simulink model "posFuzzy"  (R2015a)
settings: Solver=ode45  SolverMode=SingleTasking  StartTime=0.0  StopTime=3  RelTol=1e-3
libraries: simulink x5, fuzblock x4, simulink_extras x3
settings Model: CovMetricSettings=dwe  CovHtmlReporting=off  covSaveCumulativeToWorkspaceVar=off  CovSaveSingleToWorkspaceVar=off  CovExternalEMLEnable=on  Creator=brand  LastModifiedBy=brand
settings DataIOCC: LimitDataPoints=off  SaveFormat=Dataset
settings DebuggingCC: SFUnexpectedBacktrackingDiag=error  SFNoUnconditionalDefaultTransitionDiag=error
settings HardwareCC: ProdBitPerPointer=64  ProdLargestAtomicFloat=Float  ProdIntDivRoundTo=Zero  ProdEndianess=LittleEndian  ProdHWDeviceType=Specified
settings ModelReferenceCC: PropagateSignalLabelsOutOfModel=on
settings GRTTargetCC: TargetLangStandard=C99 (ISO)  GeneratePreprocessorConditionals=Use local settings

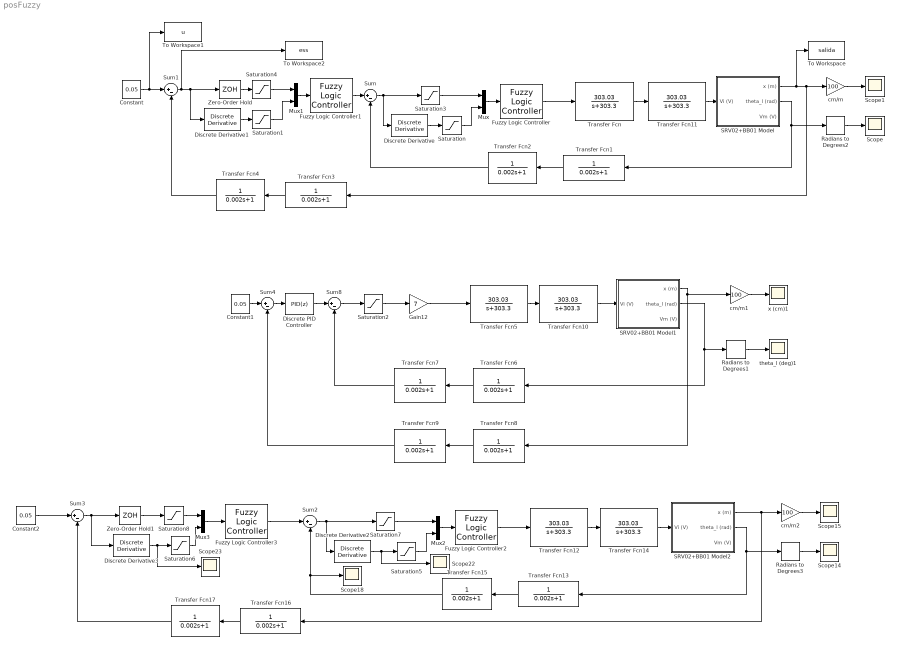
== system posFuzzy ==
  Constant : Constant  Value=0.05
  Constant1 : Constant  Value=0.05
  Constant2 : Constant  Value=0.05
  Discrete Derivative{,1..3} (4 alike) : simulink/Discrete/Discrete Derivative  gainval=1.0  ICPrevScaledInput=0.0  OutMin=[]  OutMax=[]  OutDataType=fixdt(1, 16)  OutScaling=2^-10  DoSatur=off
  Discrete PID Controller : simulink/Continuous/PID Controller  Controller=PID  TimeDomain=Discrete-time  SampleTime=12e-3  IntegratorMethod=Forward Euler  FilterMethod=Forward Euler  Form=Parallel  UseFilter=on  ControllerParametersSource=internal  P=12  I=0  D=6.5  N=100  InitialConditionSource=internal  InitialConditionForIntegrator=0  InitialConditionForFilter=0  ExternalReset=none  LimitOutput=off  UpperSaturationLimit=inf  LowerSaturationLimit=-inf  LinearizeAsGain=off  AntiWindupMode=none  Kb=1  TrackingMode=off  Kt=1  PParamMin=[]  PParamMax=[]  IParamMin=[]  IParamMax=[]  DParamMin=[]  DParamMax=[]  NParamMin=[]  NParamMax=[]  KbParamMin=[]  KbParamMax=[]  KtParamMin=[]  KtParamMax=[]  POutMin=[]  POutMax=[]  IOutMin=[]  IOutMax=[]  DOutMin=[]  DOutMax=[]  NOutMin=[]  NOutMax=[]  KbOutMin=[]  KbOutMax=[]  KtOutMin=[]  KtOutMax=[]  IntegratorOutMin=[]  IntegratorOutMax=[]  FilterOutMin=[]  FilterOutMax=[]  SumOutMin=[]  SumOutMax=[]  SumI1OutMin=[]  SumI1OutMax=[]  SumI2OutMin=[]  SumI2OutMax=[]  SumI3OutMin=[]  SumI3OutMax=[]  SumDOutMin=[]  SumDOutMax=[]  SaturationOutMin=[]  SaturationOutMax=[]  IntegratorContinuousStateAttributes=''  IntegratorStateMustResolveToSignalObject=off  IntegratorRTWStateStorageClass=Auto  FilterContinuousStateAttributes=''  FilterStateMustResolveToSignalObject=off  FilterRTWStateStorageClass=Auto  DifferentiatorICPrevScaledInput=0  DifferentiatorOutMin=[]  DifferentiatorOutMax=[]
  Fuzzy Logic Controller : fuzblock/Fuzzy Logic  Controller  FIS=angulov6unicamf
  Fuzzy Logic Controller1 : fuzblock/Fuzzy Logic  Controller  FIS=posicion8unicamf
  Fuzzy Logic Controller2 : fuzblock/Fuzzy Logic  Controller  FIS=angulov6unicamf
  Fuzzy Logic Controller3 : fuzblock/Fuzzy Logic  Controller  FIS=optipos3h
  Gain12 : Gain  Gain=7
  Mux{,1..3} (4 alike) : Mux  Inputs=2
  Radians to Degrees1 : simulink_extras/Transformations/Radians to Degrees
  Radians to Degrees2 : simulink_extras/Transformations/Radians to Degrees
  Radians to Degrees3 : simulink_extras/Transformations/Radians to Degrees
  SRV02+BB01 Model : Subsystem
  SRV02+BB01 Model1 : Subsystem
  SRV02+BB01 Model2 : Subsystem
  Saturation : Saturate  UpperLimit=5  LowerLimit=-5
  Saturation1 : Saturate  UpperLimit=20  LowerLimit=-20
  Saturation2 : Saturate  UpperLimit=0.76  LowerLimit=-0.76
  Saturation3 : Saturate  UpperLimit=0.785  LowerLimit=-0.785
  Saturation4 : Saturate  UpperLimit=0.2  LowerLimit=-0.2
  Saturation5 : Saturate  UpperLimit=5  LowerLimit=-5
  Saturation6 : Saturate  UpperLimit=20  LowerLimit=-20
  Saturation7 : Saturate  UpperLimit=0.785  LowerLimit=-0.785
  Saturation8 : Saturate  UpperLimit=0.2  LowerLimit=-0.2
  Scope{,1,14..15,18,22..23} (7 alike) : Scope
      Scope settings: TimeRange=auto  MaxDataPoints=5000  SaveToWorkspace=off  SaveName=ScopeData  YMin=-21.83998  YMax=37.02972  SampleTime=-1
      Scope1 settings: TimeRange=auto  MaxDataPoints=5000  SaveName=difuso  YMin=-0.64374  YMax=5.79369  SampleTime=-1  DataFormat=Array
      Scope14 settings: TimeRange=auto  MaxDataPoints=5000  SaveToWorkspace=off  SaveName=ScopeData6  YMin=-21.83998  YMax=37.02972  SampleTime=-1
      Scope15 settings: TimeRange=auto  MaxDataPoints=5000  SaveName=optifuzzy  YMin=-0.63086  YMax=5.67771  SampleTime=-1  DataFormat=Array
      Scope18 settings: TimeRange=auto  MaxDataPoints=5000  SaveToWorkspace=off  SaveName=ScopeData9  YMin=-0.41326  YMax=0.50458  SampleTime=-1
      Scope22 settings: TimeRange=auto  MaxDataPoints=5000  SaveToWorkspace=off  SaveName=ScopeData13  YMin=-11.56987  YMax=45.64384  SampleTime=-1
      Scope23 settings: TimeRange=auto  MaxDataPoints=5000  SaveToWorkspace=off  SaveName=ScopeData14  YMin=-0.00059  YMax=-0.00038  SampleTime=-1
  Sum{,1..4,8} (6 alike) : Sum  Inputs=|+-
  To Workspace : ToWorkspace  VariableName=salida  SaveFormat=Structure With Time  SampleTime=-1
  To Workspace1 : ToWorkspace  VariableName=u  SampleTime=-1
  To Workspace2 : ToWorkspace  VariableName=ess  SampleTime=-1
  Transfer Fcn{,5,10..12,14} (6 alike) : TransferFcn  Numerator=[303.03]  Denominator=[1 303.3]
  Transfer Fcn{1..4,6..9,13,15..17} (12 alike) : TransferFcn  Denominator=[0.002 1]
  Zero-Order Hold : ZeroOrderHold  SampleTime=12e-3
  Zero-Order Hold1 : ZeroOrderHold  SampleTime=12e-3
  cm/m : Gain  Gain=100
  cm/m1 : Gain  Gain=100
  cm/m2 : Gain  Gain=100
  theta_l (deg)1 : Scope
      settings: TimeRange=0.2  MaxDataPoints=5000  SaveName=ScopeData8  YMin=-25.81025  YMax=4.78166  SampleTime=-1  DataFormat=Array
  x (cm)1 : Scope
      settings: TimeRange=10  MaxDataPoints=5000  SaveName=convencional  YMin=-0.70041  YMax=6.30365  SampleTime=-1  DataFormat=Array
  wires:
  Mux/1 -> Fuzzy Logic Controller/1
  Sum/1 -> Saturation3/1, Discrete Derivative/1
  Fuzzy Logic Controller/1 -> Transfer Fcn/1
  Transfer Fcn1/1 -> Transfer Fcn2/1
  SRV02+BB01 Model/2(theta_l (rad)) -> Radians to Degrees2/1, Transfer Fcn1/1
  Radians to Degrees2/1 -> Scope/1
  Fuzzy Logic Controller1/1 -> Sum/1
  Transfer Fcn3/1 -> Transfer Fcn4/1
  Transfer Fcn4/1 -> Sum1/2
  Zero-Order Hold/1 -> Saturation4/1
  Mux1/1 -> Fuzzy Logic Controller1/1
  Constant/1 -> To Workspace1/1, Sum1/1
  Discrete Derivative/1 -> Saturation/1
  Saturation/1 -> Mux/2
  Discrete Derivative1/1 -> Saturation1/1
  Saturation1/1 -> Mux1/2
  Saturation4/1 -> Mux1/1
  Transfer Fcn8/1 -> Transfer Fcn9/1
  SRV02+BB01 Model1/2(theta_l (rad)) -> Radians to Degrees1/1, Transfer Fcn6/1
  Sum8/1 -> Saturation2/1
  Saturation2/1 -> Gain12/1
  Sum4/1 -> Discrete PID Controller/1
  Constant1/1 -> Sum4/1
  Discrete PID Controller/1 -> Sum8/1
  Radians to Degrees1/1 -> theta_l (deg)1/1
  Gain12/1 -> Transfer Fcn5/1
  Transfer Fcn7/1 -> Sum8/2
  Transfer Fcn9/1 -> Sum4/2
  Transfer Fcn6/1 -> Transfer Fcn7/1
  SRV02+BB01 Model1/1(x (m)) -> cm/m1/1, Transfer Fcn8/1
  cm/m1/1 -> x (cm)1/1
  Transfer Fcn5/1 -> Transfer Fcn10/1
  Transfer Fcn10/1 -> SRV02+BB01 Model1/1(Vi (V))
  Transfer Fcn/1 -> Transfer Fcn11/1
  Saturation3/1 -> Mux/1
  Transfer Fcn11/1 -> SRV02+BB01 Model/1(Vi (V))
  Transfer Fcn2/1 -> Sum/2
  Transfer Fcn15/1 -> Sum2/2, Scope18/1
  Transfer Fcn14/1 -> SRV02+BB01 Model2/1(Vi (V))
  Saturation7/1 -> Mux2/1
  Transfer Fcn12/1 -> Transfer Fcn14/1
  Saturation8/1 -> Mux3/1
  cm/m2/1 -> Scope15/1
  Saturation6/1 -> Mux3/2
  Discrete Derivative3/1 -> Saturation6/1, Scope23/1
  Saturation5/1 -> Mux2/2
  Discrete Derivative2/1 -> Saturation5/1, Scope22/1
  Constant2/1 -> Sum3/1
  Mux3/1 -> Fuzzy Logic Controller3/1
  Zero-Order Hold1/1 -> Saturation8/1
  Transfer Fcn17/1 -> Sum3/2
  Sum3/1 -> Zero-Order Hold1/1, Discrete Derivative3/1
  SRV02+BB01 Model2/1(x (m)) -> Transfer Fcn16/1, cm/m2/1
  Fuzzy Logic Controller3/1 -> Sum2/1
  Radians to Degrees3/1 -> Scope14/1
  SRV02+BB01 Model2/2(theta_l (rad)) -> Transfer Fcn13/1, Radians to Degrees3/1
  Transfer Fcn13/1 -> Transfer Fcn15/1
  Fuzzy Logic Controller2/1 -> Transfer Fcn12/1
  Sum2/1 -> Discrete Derivative2/1, Saturation7/1
  Mux2/1 -> Fuzzy Logic Controller2/1
  Transfer Fcn16/1 -> Transfer Fcn17/1
  cm/m/1 -> Scope1/1
  Sum1/1 -> To Workspace2/1, Discrete Derivative1/1, Zero-Order Hold/1
  SRV02+BB01 Model/1(x (m)) -> To Workspace/1, cm/m/1, Transfer Fcn3/1

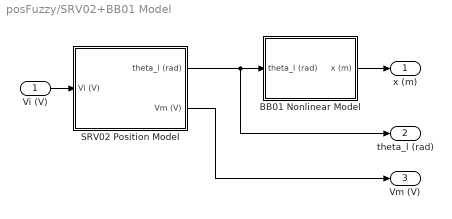
== system posFuzzy/SRV02+BB01 Model ==
  Vi (V) : Inport
  BB01 Nonlinear Model : Subsystem
  SRV02 Position Model : Subsystem
  x (m) : Outport
  theta_l (rad) : Outport  Port=2
  Vm (V) : Outport  Port=3
  wires:
  SRV02 Position Model/1(theta_l (rad)) -> BB01 Nonlinear Model/1(theta_l (rad)), theta_l (rad)/1
  BB01 Nonlinear Model/1(x (m)) -> x (m)/1
  Vi (V)/1 -> SRV02 Position Model/1(Vi (V))
  SRV02 Position Model/2(Vm (V)) -> Vm (V)/1

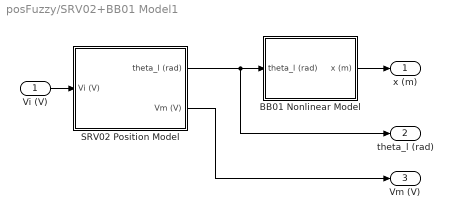
== system posFuzzy/SRV02+BB01 Model1 ==
  Vi (V) : Inport
  BB01 Nonlinear Model : Subsystem
  SRV02 Position Model : Subsystem
  x (m) : Outport
  theta_l (rad) : Outport  Port=2
  Vm (V) : Outport  Port=3
  wires:
  SRV02 Position Model/1(theta_l (rad)) -> BB01 Nonlinear Model/1(theta_l (rad)), theta_l (rad)/1
  BB01 Nonlinear Model/1(x (m)) -> x (m)/1
  Vi (V)/1 -> SRV02 Position Model/1(Vi (V))
  SRV02 Position Model/2(Vm (V)) -> Vm (V)/1

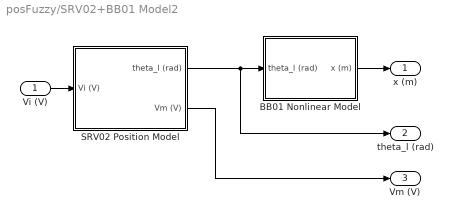
== system posFuzzy/SRV02+BB01 Model2 ==
  Vi (V) : Inport
  BB01 Nonlinear Model : Subsystem
  SRV02 Position Model : Subsystem
  x (m) : Outport
  theta_l (rad) : Outport  Port=2
  Vm (V) : Outport  Port=3
  wires:
  SRV02 Position Model/2(Vm (V)) -> Vm (V)/1
  Vi (V)/1 -> SRV02 Position Model/1(Vi (V))
  BB01 Nonlinear Model/1(x (m)) -> x (m)/1
  SRV02 Position Model/1(theta_l (rad)) -> theta_l (rad)/1, BB01 Nonlinear Model/1(theta_l (rad))

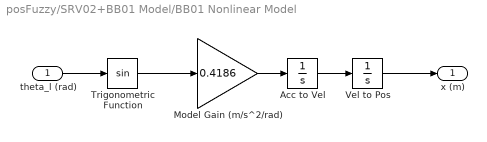
== system posFuzzy/SRV02+BB01 Model/BB01 Nonlinear Model ==
  theta_l (rad) : Inport
  Acc to Vel : Integrator
  Model Gain (m/s^2/rad) : Gain  Gain=0.4186
  Trigonometric Function : Trigonometry
  Vel to Pos : Integrator
  x (m) : Outport
  wires:
  theta_l (rad)/1 -> Trigonometric Function/1
  Vel to Pos/1 -> x (m)/1
  Model Gain (m/s^2/rad)/1 -> Acc to Vel/1
  Acc to Vel/1 -> Vel to Pos/1
  Trigonometric Function/1 -> Model Gain (m/s^2/rad)/1

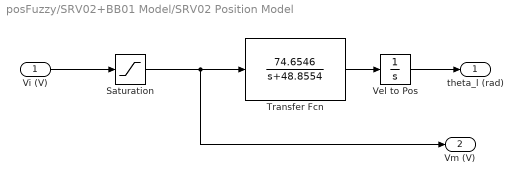
== system posFuzzy/SRV02+BB01 Model/SRV02 Position Model ==
  Vi (V) : Inport
  Saturation : Saturate  UpperLimit=5  LowerLimit=-5
  Transfer Fcn : TransferFcn  Numerator=[74.6546]  Denominator=[1 48.8554]
  Vel to Pos : Integrator
  theta_l (rad) : Outport
  Vm (V) : Outport  Port=2
  wires:
  Transfer Fcn/1 -> Vel to Pos/1
  Vel to Pos/1 -> theta_l (rad)/1
  Saturation/1 -> Vm (V)/1, Transfer Fcn/1
  Vi (V)/1 -> Saturation/1

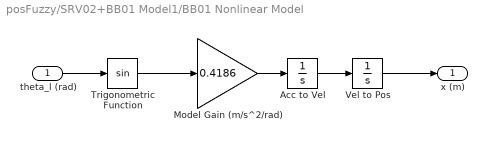
== system posFuzzy/SRV02+BB01 Model1/BB01 Nonlinear Model ==
  theta_l (rad) : Inport
  Acc to Vel : Integrator
  Model Gain (m/s^2/rad) : Gain  Gain=0.4186
  Trigonometric Function : Trigonometry
  Vel to Pos : Integrator
  x (m) : Outport
  wires:
  theta_l (rad)/1 -> Trigonometric Function/1
  Vel to Pos/1 -> x (m)/1
  Model Gain (m/s^2/rad)/1 -> Acc to Vel/1
  Acc to Vel/1 -> Vel to Pos/1
  Trigonometric Function/1 -> Model Gain (m/s^2/rad)/1

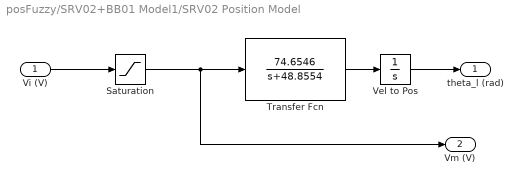
== system posFuzzy/SRV02+BB01 Model1/SRV02 Position Model ==
  Vi (V) : Inport
  Saturation : Saturate  UpperLimit=5  LowerLimit=-5
  Transfer Fcn : TransferFcn  Numerator=[74.6546]  Denominator=[1 48.8554]
  Vel to Pos : Integrator
  theta_l (rad) : Outport
  Vm (V) : Outport  Port=2
  wires:
  Transfer Fcn/1 -> Vel to Pos/1
  Vel to Pos/1 -> theta_l (rad)/1
  Saturation/1 -> Vm (V)/1, Transfer Fcn/1
  Vi (V)/1 -> Saturation/1

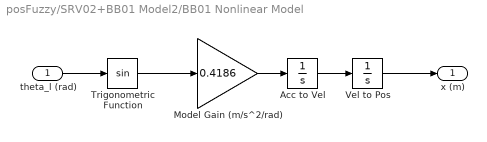
== system posFuzzy/SRV02+BB01 Model2/BB01 Nonlinear Model ==
  theta_l (rad) : Inport
  Acc to Vel : Integrator
  Model Gain (m/s^2/rad) : Gain  Gain=0.4186
  Trigonometric Function : Trigonometry
  Vel to Pos : Integrator
  x (m) : Outport
  wires:
  Trigonometric Function/1 -> Model Gain (m/s^2/rad)/1
  Acc to Vel/1 -> Vel to Pos/1
  Model Gain (m/s^2/rad)/1 -> Acc to Vel/1
  Vel to Pos/1 -> x (m)/1
  theta_l (rad)/1 -> Trigonometric Function/1

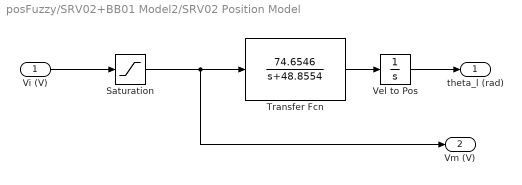
== system posFuzzy/SRV02+BB01 Model2/SRV02 Position Model ==
  Vi (V) : Inport
  Saturation : Saturate  UpperLimit=5  LowerLimit=-5
  Transfer Fcn : TransferFcn  Numerator=[74.6546]  Denominator=[1 48.8554]
  Vel to Pos : Integrator
  theta_l (rad) : Outport
  Vm (V) : Outport  Port=2
  wires:
  Vi (V)/1 -> Saturation/1
  Saturation/1 -> Transfer Fcn/1, Vm (V)/1
  Vel to Pos/1 -> theta_l (rad)/1
  Transfer Fcn/1 -> Vel to Pos/1
